simulink library "Simscape_Gimbals__Lib"  (R2025b)
settings: Solver=VariableStepAuto  StartTime=0.0  StopTime=10.0  RelTol=1e-3
undefined symbols (not defined in the file or in its folder): axisCmdType, baseAccEcho, baseRatesEcho, cmdTypes, dt, Motion, nFrames, Support, tFrame, tMotion, yawVec
libraries: nesl_utility x40, fl_lib x18, $bdroot x9, sm_lib x6, simulink_extras x6, simulink x1
(part 1 of 2)
settings Model: Creator=leoni  LastModifiedBy=Leonid

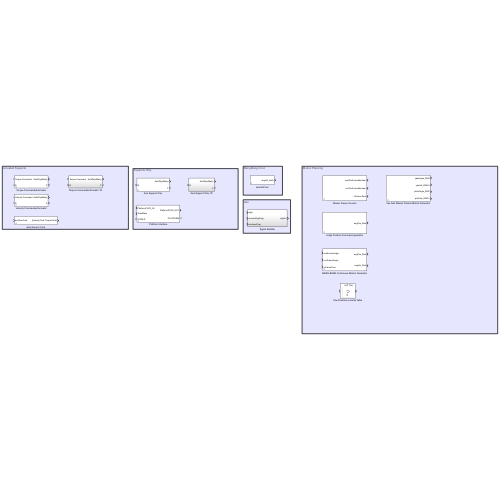
[thumbnail: Simulink's stored preview of the top-level diagram]
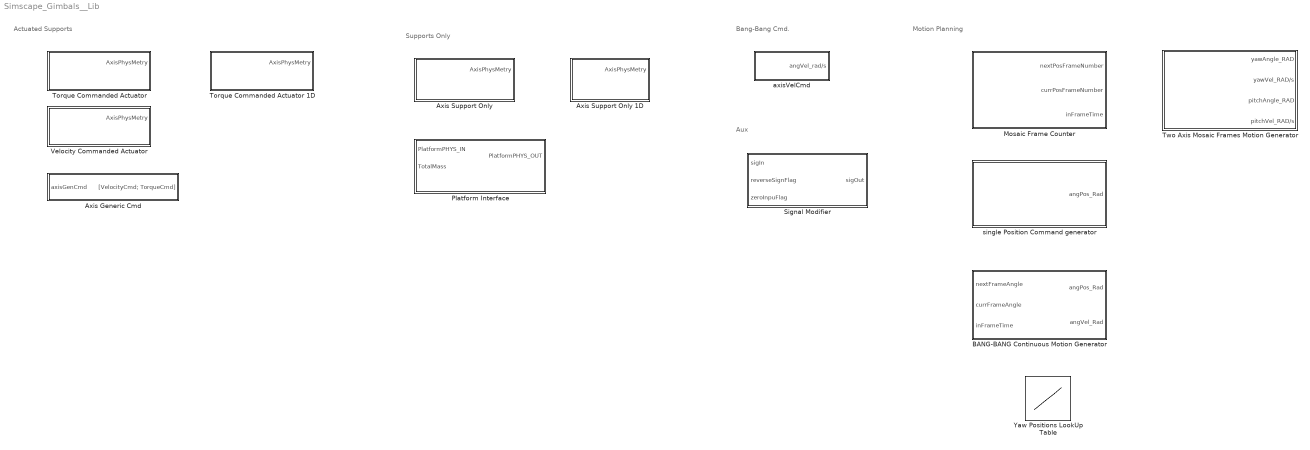
== system Simscape_Gimbals__Lib ==
  note: Aux
  note: Bang-Bang Cmd.
  note: Supports Only
  note: Actuated Supports
  note: Motion Planning
  Axis Generic Cmd : Subsystem  mask{AxisCmdType=axisCmdType}
      mask prompts: AxisCmdType "Axis Command Type"
  Axis Support Only : Subsystem  mask{bearingProps=0, noDist=on}
      mask prompts: bearingProps "Bearing Properties"; noDist "No Disturbances"
  Axis Support Only 1D : Subsystem
  BANG-BANG Continuous Motion Generator : Subsystem  mask{tMotion=tMotion, tFrame=tFrame}
      mask prompts: tMotion "Motion Time [s]"; tFrame "Frame Time [s]"
      mask DialogControl ParameterGroupVar Prompt: Bang-Bang
  Mosaic Frame Counter : Subsystem  mask{tFrame=tFrame, dt=dt, nFrames=0}
      mask prompts: tFrame "Frame time [s]"; dt "Sim resolution [s]"; nFrames "Number of Frames"
  Platform Interface : Subsystem  mask{mappingX=X, reverseX=off, mappingY=X, reverseY=off, mappingZ=X, reverseZ=off, noBaseMotion=off}
      mask prompts: mappingX "Map System X to World"; reverseX "Reverse X Direction"; mappingY "Map System Y to World"; reverseY "Reverse Y Direction"; mappingZ "Map System Z to World"; reverseZ "Reverse Z Direction"; noBaseMotion "No Base Motion"
      mask DialogControl ParameterGroupVar Prompt: CS MAPPING
      mask DialogControl Container3 Prompt: Simplifications
  Signal Modifier : Subsystem
  Torque Commanded Actuator : Subsystem  mask{bearingProps=0, harnessConstant=0, noDist=on}
      mask prompts: bearingProps "Bearing Properties"; harnessConstant "Harness Constant [mNm/rad]"; noDist "No Disturbances"
  Torque Commanded Actuator 1D : Subsystem
  Two Axis Mosaic Frames Motion Generator : Subsystem  mask{dt=0, tFrame=0, tMotion=0, nFrames=0, yawVec_DEG=0, pitchVec_DEG=0}
      mask prompts: dt "Simulation Time Resolution [s]"; tFrame "Single Frame Duration [s]"; tMotion "In Frame Motion Duration [s]"; nFrames "Total Number Of Frames"; yawVec_DEG "Yaw Axis Angle Sequence [DEG}"; pitchVec_DEG "PitchAxis Angle Sequence [DEG]"
      mask DialogControl ParameterGroupVar Prompt: Motion Time Properties
      mask DialogControl Container3 Prompt: Motion Angles
  Velocity Commanded Actuator : Subsystem  mask{bearingProps=0, harnessConstant=0}
      mask prompts: bearingProps "Bearing Properties"; harnessConstant "Harness Constant [mNm/rad]"
  Yaw Positions LookUp Table : Lookup_n-D  NumberOfTableDimensions=1  BreakpointsForDimension1=1:nFrames  Table=yawVec  InternalRulePriority=Speed  RndMeth=Simplest
  axisVelCmd : Subsystem  mask{travel=0.0, tMotion=0.0, tStart=0}
      mask prompts: travel "Travel Angle [deg]"; tMotion "Motion Duration [ms]"; tStart "Starting Time [s]"
      mask DialogControl ParameterGroupVar Prompt: Bang-Bang
  single Position Command generator : Subsystem  mask{Angle=15, Time=70}
      mask prompts: Angle "Travel Angle [deg]"; Time "Travel Time [ms]"
      mask DialogControl ParameterGroupVar Prompt: Bang-Bang

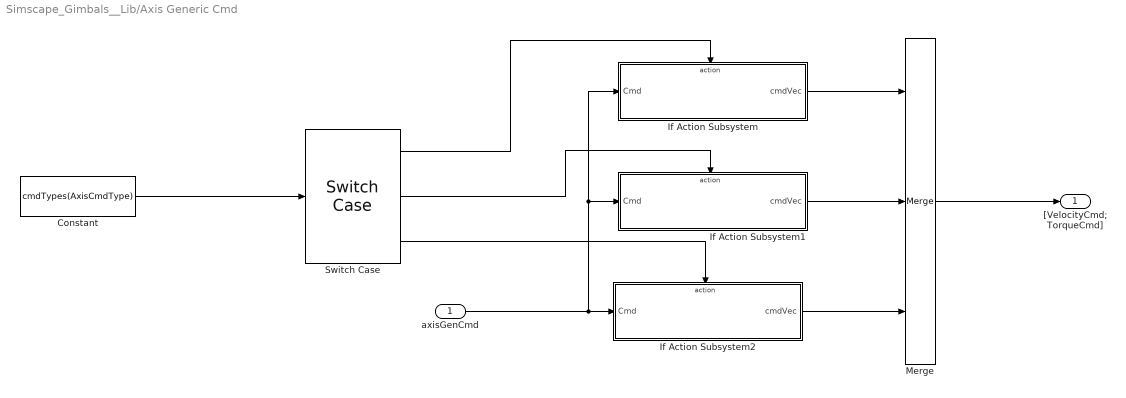
== system Simscape_Gimbals__Lib/Axis Generic Cmd ==
  axisGenCmd : Inport
  Constant : Constant  Value=cmdTypes(AxisCmdType)  OutDataTypeStr=Enum: cmdTypes
  If Action Subsystem : Subsystem  TreatAsAtomicUnit=on
  If Action Subsystem1 : Subsystem  TreatAsAtomicUnit=on
  If Action Subsystem2 : Subsystem  TreatAsAtomicUnit=on
  Merge : Merge  Inputs=3
  Switch Case : SwitchCase  CaseConditions={cmdTypes(1), cmdTypes(2)}
  "[VelocityCmd; TorqueCmd]" : Outport
  wires:
  Switch Case/1 -> If Action Subsystem/Action
  Switch Case/2 -> If Action Subsystem1/Action
  Switch Case/3 -> If Action Subsystem2/Action
  If Action Subsystem2/1(cmdVec) -> Merge/3
  If Action Subsystem1/1(cmdVec) -> Merge/2
  If Action Subsystem/1(cmdVec) -> Merge/1
  Merge/1 -> "[VelocityCmd; TorqueCmd]"/1
  axisGenCmd/1 -> If Action Subsystem/1(Cmd), If Action Subsystem1/1(Cmd), If Action Subsystem2/1(Cmd)
  Constant/1 -> Switch Case/1

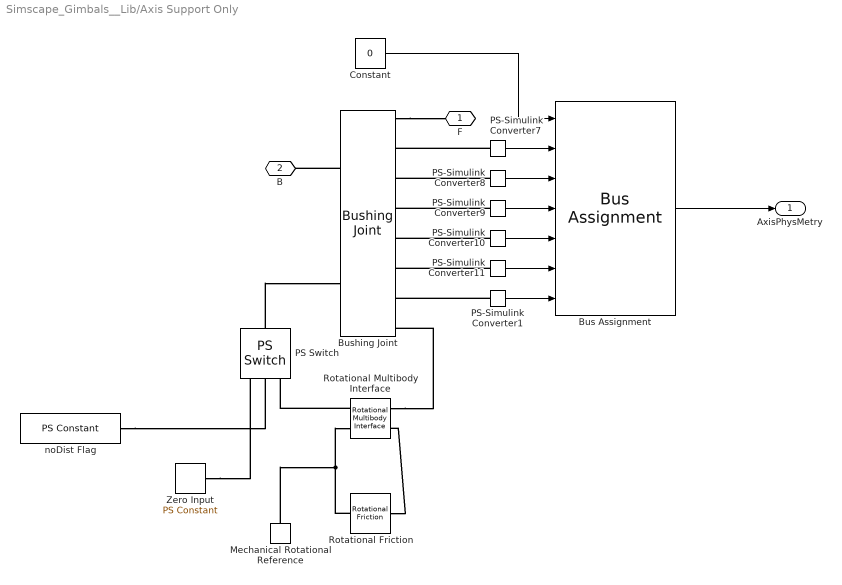
== system Simscape_Gimbals__Lib/Axis Support Only ==
  Bus Assignment : BusAssignment  AssignedSignals=Support.pX,Support.pY,Support.pZ,Support.qX,Support.qY,Motion.AxisPosition
  Bushing Joint : sm_lib/Joints/Bushing Joint  JointMode=Normal  CompositeWrenchDir=FollowerOnBase  CompositeWrenchFrame=BaseFrame  SenseConstraintForce=off  SenseConstraintTorque=off  SenseTotalForce=off  SenseTotalTorque=off  PxPositionTargetSpecify=off  PxPositionTargetPriority=High  PxPositionTargetValue=0  PxPositionTargetValueUnits=m  PxVelocityTargetSpecify=off  PxVelocityTargetPriority=High  PxVelocityTargetValue=0  PxVelocityTargetValueUnits=m/s  PxEquilibriumPosition=0.0  PxEquilibriumPositionUnits=mm  PxSpringStiffness=bearingProps.Krad  PxSpringStiffnessUnits=N/mm  PxDampingCoefficient=bearingProps.Crad  PxDampingCoefficientUnits=N/(m/s)  PxLowerLimitSpecify=off  PxLowerLimitBound=-1  PxLowerLimitBoundUnits=m  PxLowerLimitStiffness=1e6  PxLowerLimitStiffnessUnits=N/m  PxLowerLimitDamping=1e3  PxLowerLimitDampingUnits=N/(m/s)  PxLowerLimitTransitionRegionWidth=1e-4  PxLowerLimitTransitionRegionWidthUnits=m  PxUpperLimitSpecify=off  PxUpperLimitBound=1  PxUpperLimitBoundUnits=m  PxUpperLimitStiffness=1e6  PxUpperLimitStiffnessUnits=N/m  PxUpperLimitDamping=1e3  PxUpperLimitDampingUnits=N/(m/s)  PxUpperLimitTransitionRegionWidth=1e-4  PxUpperLimitTransitionRegionWidthUnits=m  PxTorqueActuationMode=NoTorque  PxMotionActuationMode=ComputedMotion  PxSensePosition=on  PxSenseVelocity=off  PxSenseAcceleration=off  PxSenseTorqueForce=off  PxSenseLowerLimitTorqueForce=off  PxSenseUpperLimitTorqueForce=off  PyPositionTargetSpecify=off  PyPositionTargetPriority=High  PyPositionTargetValue=0  PyPositionTargetValueUnits=m  PyVelocityTargetSpecify=off  PyVelocityTargetPriority=High  PyVelocityTargetValue=0  PyVelocityTargetValueUnits=m/s  PyEquilibriumPosition=0  PyEquilibriumPositionUnits=m  PySpringStiffness=bearingProps.Krad  PySpringStiffnessUnits=N/mm  PyDampingCoefficient=bearingProps.Crad  PyDampingCoefficientUnits=N/(m/s)  PyLowerLimitSpecify=off  PyLowerLimitBound=-1  PyLowerLimitBoundUnits=m  PyLowerLimitStiffness=1e6  PyLowerLimitStiffnessUnits=N/m  PyLowerLimitDamping=1e3  PyLowerLimitDampingUnits=N/(m/s)  PyLowerLimitTransitionRegionWidth=1e-4  PyLowerLimitTransitionRegionWidthUnits=m  PyUpperLimitSpecify=off  PyUpperLimitBound=1  PyUpperLimitBoundUnits=m  PyUpperLimitStiffness=1e6  PyUpperLimitStiffnessUnits=N/m  PyUpperLimitDamping=1e3  PyUpperLimitDampingUnits=N/(m/s)  PyUpperLimitTransitionRegionWidth=1e-4  PyUpperLimitTransitionRegionWidthUnits=m  PyTorqueActuationMode=NoTorque  PyMotionActuationMode=ComputedMotion  PySensePosition=on  PySenseVelocity=off  PySenseAcceleration=off  PySenseTorqueForce=off  PySenseLowerLimitTorqueForce=off  PySenseUpperLimitTorqueForce=off  PzPositionTargetSpecify=off  PzPositionTargetPriority=High  PzPositionTargetValue=0  PzPositionTargetValueUnits=m  PzVelocityTargetSpecify=off  PzVelocityTargetPriority=High  PzVelocityTargetValue=0  PzVelocityTargetValueUnits=m/s  PzEquilibriumPosition=0.0  PzEquilibriumPositionUnits=mm  PzSpringStiffness=bearingProps.Kax  PzSpringStiffnessUnits=N/mm  PzDampingCoefficient=bearingProps.Cax  PzDampingCoefficientUnits=N/(m/s)  PzLowerLimitSpecify=off  PzLowerLimitBound=-1  PzLowerLimitBoundUnits=m  PzLowerLimitStiffness=1e6  PzLowerLimitStiffnessUnits=N/m  PzLowerLimitDamping=1e3  PzLowerLimitDampingUnits=N/(m/s)  PzLowerLimitTransitionRegionWidth=1e-4  PzLowerLimitTransitionRegionWidthUnits=m  PzUpperLimitSpecify=off  PzUpperLimitBound=1  PzUpperLimitBoundUnits=m  PzUpperLimitStiffness=1e6  PzUpperLimitStiffnessUnits=N/m  PzUpperLimitDamping=1e3  PzUpperLimitDampingUnits=N/(m/s)  PzUpperLimitTransitionRegionWidth=1e-4  PzUpperLimitTransitionRegionWidthUnits=m  PzTorqueActuationMode=NoTorque  PzMotionActuationMode=ComputedMotion  PzSensePosition=on  PzSenseVelocity=off  PzSenseAcceleration=off  PzSenseTorqueForce=off  PzSenseLowerLimitTorqueForce=off  PzSenseUpperLimitTorqueForce=off  RxPositionTargetSpecify=off  RxPositionTargetPriority=High  RxPositionTargetValue=0  RxPositionTargetValueUnits=deg  RxVelocityTargetSpecify=off  RxVelocityTargetPriority=High  RxVelocityTargetValue=0  RxVelocityTargetValueUnits=deg/s  RxEquilibriumPosition=0.0  RxEquilibriumPositionUnits=deg  RxSpringStiffness=bearingProps.Kang  RxSpringStiffnessUnits=N*m/rad  RxDampingCoefficient=bearingProps.Cang  RxDampingCoefficientUnits=N*m*s/rad  RxLowerLimitSpecify=off  RxLowerLimitBound=-90  RxLowerLimitBoundUnits=deg  RxLowerLimitStiffness=1e4  RxLowerLimitStiffnessUnits=N*m/deg  RxLowerLimitDamping=10  RxLowerLimitDampingUnits=N*m/(deg/s)  RxLowerLimitTransitionRegionWidth=0.1  RxLowerLimitTransitionRegionWidthUnits=deg  RxUpperLimitSpecify=off  RxUpperLimitBound=90  RxUpperLimitBoundUnits=deg  RxUpperLimitStiffness=1e4  RxUpperLimitStiffnessUnits=N*m/deg  RxUpperLimitDamping=10  RxUpperLimitDampingUnits=N*m/(deg/s)  RxUpperLimitTransitionRegionWidth=0.1  RxUpperLimitTransitionRegionWidthUnits=deg  RxTorqueActuationMode=NoTorque  RxMotionActuationMode=ComputedMotion  RxSensePosition=on  RxSenseVelocity=off  RxSenseAcceleration=off  RxSenseTorqueForce=off  RxSenseLowerLimitTorqueForce=off  RxSenseUpperLimitTorqueForce=off  RyPositionTargetSpecify=off  RyPositionTargetPriority=High  RyPositionTargetValue=0  RyPositionTargetValueUnits=deg  RyVelocityTargetSpecify=off  RyVelocityTargetPriority=High  RyVelocityTargetValue=0  RyVelocityTargetValueUnits=deg/s  RyEquilibriumPosition=0.0  RyEquilibriumPositionUnits=deg  RySpringStiffness=bearingProps.Kang  RySpringStiffnessUnits=N*m/rad  RyDampingCoefficient=bearingProps.Cang  RyDampingCoefficientUnits=N*m*s/rad  RyLowerLimitSpecify=off  RyLowerLimitBound=-90  RyLowerLimitBoundUnits=deg  RyLowerLimitStiffness=1e4  RyLowerLimitStiffnessUnits=N*m/deg  RyLowerLimitDamping=10  RyLowerLimitDampingUnits=N*m/(deg/s)  RyLowerLimitTransitionRegionWidth=0.1  RyLowerLimitTransitionRegionWidthUnits=deg  RyUpperLimitSpecify=off  RyUpperLimitBound=90  RyUpperLimitBoundUnits=deg  RyUpperLimitStiffness=1e4  RyUpperLimitStiffnessUnits=N*m/deg  RyUpperLimitDamping=10  RyUpperLimitDampingUnits=N*m/(deg/s)  RyUpperLimitTransitionRegionWidth=0.1  RyUpperLimitTransitionRegionWidthUnits=deg  RyTorqueActuationMode=NoTorque  RyMotionActuationMode=ComputedMotion  RySensePosition=on  RySenseVelocity=off  RySenseAcceleration=off  RySenseTorqueForce=off  RySenseLowerLimitTorqueForce=off  RySenseUpperLimitTorqueForce=off  RzPositionTargetSpecify=off  RzPositionTargetPriority=High  RzPositionTargetValue=0  RzPositionTargetValueUnits=deg  RzVelocityTargetSpecify=off  RzVelocityTargetPriority=High  RzVelocityTargetValue=0  RzVelocityTargetValueUnits=deg/s  RzEquilibriumPosition=0  RzEquilibriumPositionUnits=deg  RzSpringStiffness=0  RzSpringStiffnessUnits=N*m/deg  RzDampingCoefficient=0  RzDampingCoefficientUnits=N*m/(deg/s)  RzLowerLimitSpecify=off  RzLowerLimitBound=-90  RzLowerLimitBoundUnits=deg  RzLowerLimitStiffness=1e4  RzLowerLimitStiffnessUnits=N*m/deg  RzLowerLimitDamping=10  RzLowerLimitDampingUnits=N*m/(deg/s)  RzLowerLimitTransitionRegionWidth=0.1  RzLowerLimitTransitionRegionWidthUnits=deg  RzUpperLimitSpecify=off  RzUpperLimitBound=90  RzUpperLimitBoundUnits=deg  RzUpperLimitStiffness=1e4  RzUpperLimitStiffnessUnits=N*m/deg  RzUpperLimitDamping=10  RzUpperLimitDampingUnits=N*m/(deg/s)  RzUpperLimitTransitionRegionWidth=0.1  RzUpperLimitTransitionRegionWidthUnits=deg  RzTorqueActuationMode=InputTorque  RzMotionActuationMode=ComputedMotion  RzSensePosition=on  RzSenseVelocity=on  RzSenseAcceleration=off  RzSenseTorqueForce=off  RzSenseLowerLimitTorqueForce=off  RzSenseUpperLimitTorqueForce=off
  Constant : Constant  Value=0  OutDataTypeStr=Bus: AxisMetry
  Mechanical Rotational Reference : fl_lib/Mechanical/Rotational Elements/Mechanical Rotational Reference
  PS Switch : fl_lib/Physical Signals/Nonlinear Operators/PS Switch  Threshold=0.5  ZeroCross=true
      settings: InternalSimscapePortConfiguration="{\"Bottom\":[],\"Left\":[{\"id\":\"I1\",\"label\":\"\",\"type\":\"input\"},{\"id\":\"I2\",\"label\":\"\",\"type\":\"input\"},{\"id\":\"I3\",\"label\":\"\",\"type\":\"input\"}],\"Right\":[{\"id\":\"O\",\"label\":\"\",\"type\":\"output\"}],\"Top\":[]}"
  PS-Simulink Converter1 : nesl_utility/PS-Simulink Converter  PhysicalDomain=network_engine_domain  SubClassName=ps_output  LeftPortType=input  RightPortType=output  PseudoPeriodic=off  Frequencies=[]  VectorFormat=inherit  Unit=rad  AffineConversion=off
  PS-Simulink Converter10 : nesl_utility/PS-Simulink Converter  PhysicalDomain=network_engine_domain  SubClassName=ps_output  LeftPortType=input  RightPortType=output  PseudoPeriodic=off  Frequencies=[]  VectorFormat=inherit  Unit=rad  AffineConversion=off
  PS-Simulink Converter11 : nesl_utility/PS-Simulink Converter  PhysicalDomain=network_engine_domain  SubClassName=ps_output  LeftPortType=input  RightPortType=output  PseudoPeriodic=off  Frequencies=[]  VectorFormat=inherit  Unit=rad  AffineConversion=off
  PS-Simulink Converter7 : nesl_utility/PS-Simulink Converter  PhysicalDomain=network_engine_domain  SubClassName=ps_output  LeftPortType=input  RightPortType=output  PseudoPeriodic=off  Frequencies=[]  VectorFormat=inherit  Unit=m  AffineConversion=off
  PS-Simulink Converter8 : nesl_utility/PS-Simulink Converter  PhysicalDomain=network_engine_domain  SubClassName=ps_output  LeftPortType=input  RightPortType=output  PseudoPeriodic=off  Frequencies=[]  VectorFormat=inherit  Unit=m  AffineConversion=off
  PS-Simulink Converter9 : nesl_utility/PS-Simulink Converter  PhysicalDomain=network_engine_domain  SubClassName=ps_output  LeftPortType=input  RightPortType=output  PseudoPeriodic=off  Frequencies=[]  VectorFormat=inherit  Unit=m  AffineConversion=off
  Rotational Friction : fl_lib/Mechanical/Rotational Elements/Rotational Friction  brkwy_trq=bearingProps.Tf*1.4 m*mN  brkwy_vel=0.1 rad/s  Col_trq=bearingProps.Tf m*mN  visc_coef=0.0 N*m*s/rad  w_specify=off  w_priority=None  w=0 rad/s  w_nominal_specify=off  w_nominal_value=1  w_nominal_unit=rad/s  t_specify=off  t_priority=None  t=0 N*m  t_nominal_specify=off  t_nominal_value=1  t_nominal_unit=N*m
  Rotational Multibody Interface : fl_lib/Mechanical/Multibody Interfaces/Rotational Multibody Interface
  Zero Input : fl_lib/Physical Signals/Sources/PS Constant  constant=0 N*m
  noDist Flag : fl_lib/Physical Signals/Sources/PS Constant  constant=noDist
  F : PMIOPort  Side=Right
  B : PMIOPort  Port=2  Side=Left
  AxisPhysMetry : Outport
  wires:
  Constant/1 -> Bus Assignment/1
  Bus Assignment/1 -> AxisPhysMetry/1
  PS-Simulink Converter9/1 -> Bus Assignment/4
  PS-Simulink Converter10/1 -> Bus Assignment/5
  PS-Simulink Converter11/1 -> Bus Assignment/6
  PS-Simulink Converter8/1 -> Bus Assignment/3
  PS-Simulink Converter7/1 -> Bus Assignment/2
  PS-Simulink Converter1/1 -> Bus Assignment/7
  connections:
  Rotational Friction/LConn1 -- Rotational Multibody Interface/RConn2
  Mechanical Rotational Reference/LConn1 -- Rotational Friction/RConn1 -- Rotational Multibody Interface/LConn2
  PS-Simulink Converter11/LConn1 -- Bushing Joint/RConn6
  PS-Simulink Converter9/LConn1 -- Bushing Joint/RConn4
  PS-Simulink Converter10/LConn1 -- Bushing Joint/RConn5
  Rotational Multibody Interface/RConn1 -- Bushing Joint/RConn8
  PS-Simulink Converter7/LConn1 -- Bushing Joint/RConn2
  PS-Simulink Converter1/LConn1 -- Bushing Joint/RConn7
  Bushing Joint/RConn1 -- F/RConn1
  Bushing Joint/LConn1 -- B/RConn1
  PS-Simulink Converter8/LConn1 -- Bushing Joint/RConn3
  Rotational Multibody Interface/LConn1 -- PS Switch/LConn3
  PS Switch/RConn1 -- Bushing Joint/LConn2
  noDist Flag/RConn1 -- PS Switch/LConn2
  Zero Input/RConn1 -- PS Switch/LConn1

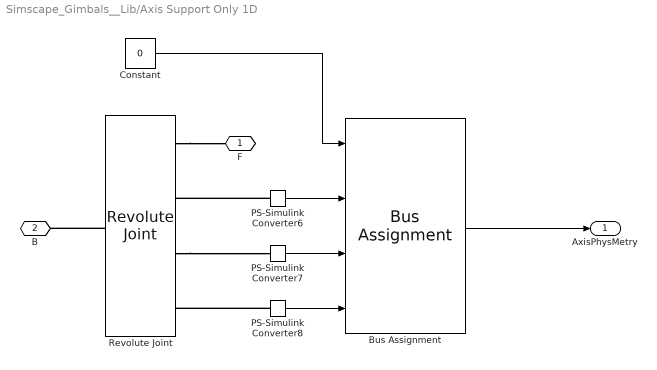
== system Simscape_Gimbals__Lib/Axis Support Only 1D ==
  Bus Assignment : BusAssignment  AssignedSignals=Motion.AxisPosition,Motion.AxisVelocity,Motion.AxisTorque
  Constant : Constant  Value=0  OutDataTypeStr=Bus: AxisMetry
  PS-Simulink Converter6 : nesl_utility/PS-Simulink Converter  PhysicalDomain=network_engine_domain  SubClassName=ps_output  LeftPortType=input  RightPortType=output  PseudoPeriodic=off  Frequencies=[]  VectorFormat=inherit  Unit=rad  AffineConversion=off
  PS-Simulink Converter7 : nesl_utility/PS-Simulink Converter  PhysicalDomain=network_engine_domain  SubClassName=ps_output  LeftPortType=input  RightPortType=output  PseudoPeriodic=off  Frequencies=[]  VectorFormat=inherit  Unit=rad/s  AffineConversion=off
  PS-Simulink Converter8 : nesl_utility/PS-Simulink Converter  PhysicalDomain=network_engine_domain  SubClassName=ps_output  LeftPortType=input  RightPortType=output  PseudoPeriodic=off  Frequencies=[]  VectorFormat=inherit  Unit=N*m  AffineConversion=off
  Revolute Joint : sm_lib/Joints/Revolute Joint  JointMode=Normal  CompositeWrenchDir=FollowerOnBase  CompositeWrenchFrame=BaseFrame  SenseConstraintForce=off  SenseConstraintTorque=off  SenseTotalForce=off  SenseTotalTorque=off  PositionTargetSpecify=off  PositionTargetPriority=High  PositionTargetValue=0  PositionTargetValueUnits=deg  VelocityTargetSpecify=off  VelocityTargetPriority=High  VelocityTargetValue=0  VelocityTargetValueUnits=deg/s  EquilibriumPosition=0  EquilibriumPositionUnits=deg  SpringStiffness=0  SpringStiffnessUnits=N*m/deg  DampingCoefficient=0  DampingCoefficientUnits=N*m/(deg/s)  LowerLimitSpecify=off  LowerLimitBound=-90  LowerLimitBoundUnits=deg  LowerLimitStiffness=1e4  LowerLimitStiffnessUnits=N*m/deg  LowerLimitDamping=10  LowerLimitDampingUnits=N*m/(deg/s)  LowerLimitTransitionRegionWidth=0.1  LowerLimitTransitionRegionWidthUnits=deg  UpperLimitSpecify=off  UpperLimitBound=90  UpperLimitBoundUnits=deg  UpperLimitStiffness=1e4  UpperLimitStiffnessUnits=N*m/deg  UpperLimitDamping=10  UpperLimitDampingUnits=N*m/(deg/s)  UpperLimitTransitionRegionWidth=0.1  UpperLimitTransitionRegionWidthUnits=deg  TorqueActuationMode=NoTorque  MotionActuationMode=ComputedMotion  SensePosition=on  SenseVelocity=on  SenseAcceleration=off  SenseTorqueForce=on  SenseLowerLimitTorqueForce=off  SenseUpperLimitTorqueForce=off
  F : PMIOPort  Side=Right
  B : PMIOPort  Port=2  Side=Left
  AxisPhysMetry : Outport
  wires:
  Constant/1 -> Bus Assignment/1
  PS-Simulink Converter6/1 -> Bus Assignment/2
  PS-Simulink Converter7/1 -> Bus Assignment/3
  PS-Simulink Converter8/1 -> Bus Assignment/4
  Bus Assignment/1 -> AxisPhysMetry/1
  connections:
  Revolute Joint/LConn1 -- B/RConn1
  Revolute Joint/RConn1 -- F/RConn1
  PS-Simulink Converter6/LConn1 -- Revolute Joint/RConn2
  Revolute Joint/RConn3 -- PS-Simulink Converter7/LConn1
  PS-Simulink Converter8/LConn1 -- Revolute Joint/RConn4

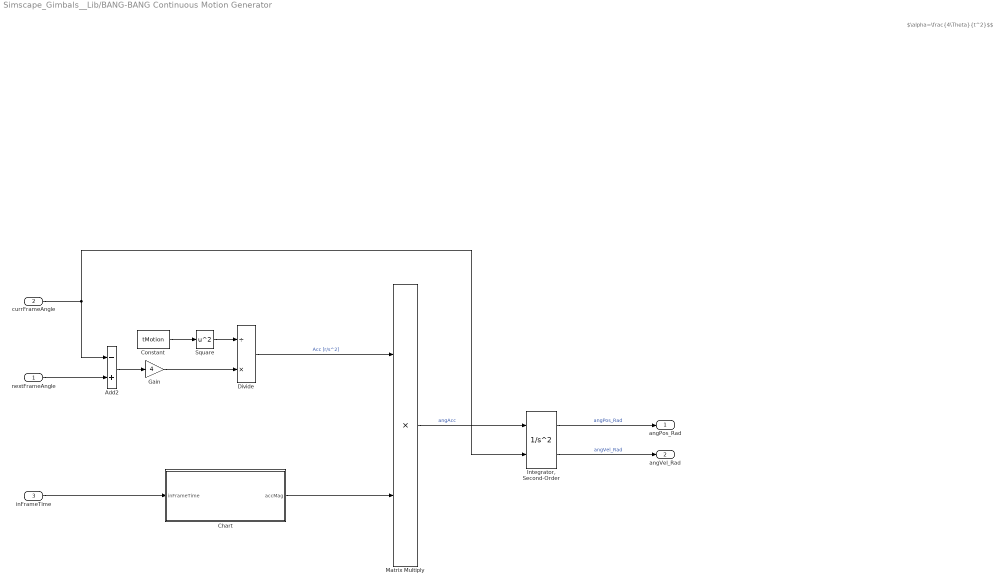
== system Simscape_Gimbals__Lib/BANG-BANG Continuous Motion Generator ==
  note: $\alpha=\frac{4\Theta}{t^2}$$
  nextFrameAngle : Inport
  currFrameAngle : Inport  Port=2
  inFrameTime : Inport  Port=3
  Add2 : Sum  Inputs=-+
  Chart : Stateflow chart  TreatAsAtomicUnit=on
  Constant : Constant  Value=tMotion
  Divide : Product  Inputs=/*
  Gain : Gain  Gain=4
  "Integrator, Second-Order" : SecondOrderIntegrator  ICSourceX=external
  Matrix Multiply : Product
  Square : Math  Operator=square
  angPos_Rad : Outport
  angVel_Rad : Outport  Port=2
  wires:
  Chart/1(accMag) -> Matrix Multiply/2
  Divide/1 -> Matrix Multiply/1  "Acc [r/s^2]"
  Matrix Multiply/1 -> "Integrator, Second-Order"/1  "angAcc"
  "Integrator, Second-Order"/1 -> angPos_Rad/1  "angPos_Rad"
  "Integrator, Second-Order"/2 -> angVel_Rad/1  "angVel_Rad"
  Constant/1 -> Square/1
  Gain/1 -> Divide/2
  Square/1 -> Divide/1
  inFrameTime/1 -> Chart/1(inFrameTime)
  Add2/1 -> Gain/1
  currFrameAngle/1 -> Add2/1, "Integrator, Second-Order"/2
  nextFrameAngle/1 -> Add2/2

== system Simscape_Gimbals__Lib/Mosaic Frame Counter ==
  Clock : Clock
  Compare To Constant : simulink/Logic and Bit Operations/Compare To Constant  relop=<=  const=dt*2  OutDataTypeStr=boolean
  Mod : Math  Operator=mod
  Triggered Subsystem : Subsystem  TreatAsAtomicUnit=on
  frame time : Constant  Value=tFrame
  nextPosFrameNumber : Outport
  currPosFrameNumber : Outport  Port=2
  inFrameTime : Outport  Port=3
  wires:
  Triggered Subsystem/1(currCMD) -> nextPosFrameNumber/1
  Mod/1 -> inFrameTime/1, Compare To Constant/1
  frame time/1 -> Mod/2
  Compare To Constant/1 -> Triggered Subsystem/Trigger
  Clock/1 -> Mod/1
  Triggered Subsystem/2(currPOS) -> currPosFrameNumber/1

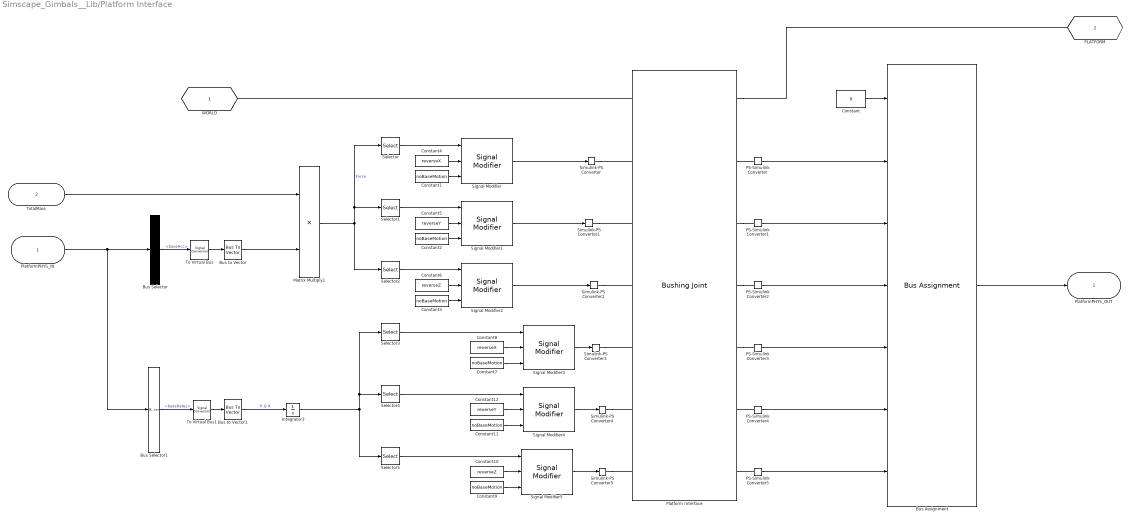
== system Simscape_Gimbals__Lib/Platform Interface ==
  PlatformPHYS_IN : Inport  OutDataTypeStr=Bus: PHYS_IN
  TotalMass : Inport  Port=2
  Bus Assignment : BusAssignment  AssignedSignals=baseAccEcho.aX,baseAccEcho.aY,baseAccEcho.aZ,baseRatesEcho.wX,baseRatesEcho.wY,baseRatesEcho.wZ
  Bus Selector : BusSelector  OutputSignals=baseAcc
  Bus Selector1 : BusSelector  OutputSignals=baseRates
  Bus to Vector : BusToVector
  Bus to Vector1 : BusToVector
  Constant : Constant  Value=0  OutDataTypeStr=Bus: PHYS_OUT  SampleTime=-1
  Constant{1..3,7,9,11} (6 alike) : Constant  Value=noBaseMotion
  Constant10 : Constant  Value=reverseZ
  Constant12 : Constant  Value=reverseY
  Constant4 : Constant  Value=reverseX
  Constant5 : Constant  Value=reverseY
  Constant6 : Constant  Value=reverseZ
  Constant8 : Constant  Value=reverseX
  Integrator3 : Integrator
  Matrix Multiply1 : Product
  PS-Simulink Converter : nesl_utility/PS-Simulink Converter  PhysicalDomain=network_engine_domain  SubClassName=ps_output  LeftPortType=input  RightPortType=output  PseudoPeriodic=off  Frequencies=[]  VectorFormat=inherit  Unit=m/s^2  AffineConversion=off
  PS-Simulink Converter1 : nesl_utility/PS-Simulink Converter  PhysicalDomain=network_engine_domain  SubClassName=ps_output  LeftPortType=input  RightPortType=output  PseudoPeriodic=off  Frequencies=[]  VectorFormat=inherit  Unit=m/s^2  AffineConversion=off
  PS-Simulink Converter2 : nesl_utility/PS-Simulink Converter  PhysicalDomain=network_engine_domain  SubClassName=ps_output  LeftPortType=input  RightPortType=output  PseudoPeriodic=off  Frequencies=[]  VectorFormat=inherit  Unit=m/s^2  AffineConversion=off
  PS-Simulink Converter3 : nesl_utility/PS-Simulink Converter  PhysicalDomain=network_engine_domain  SubClassName=ps_output  LeftPortType=input  RightPortType=output  PseudoPeriodic=off  Frequencies=[]  VectorFormat=inherit  Unit=rad/s  AffineConversion=off
  PS-Simulink Converter4 : nesl_utility/PS-Simulink Converter  PhysicalDomain=network_engine_domain  SubClassName=ps_output  LeftPortType=input  RightPortType=output  PseudoPeriodic=off  Frequencies=[]  VectorFormat=inherit  Unit=rad/s  AffineConversion=off
  PS-Simulink Converter5 : nesl_utility/PS-Simulink Converter  PhysicalDomain=network_engine_domain  SubClassName=ps_output  LeftPortType=input  RightPortType=output  PseudoPeriodic=off  Frequencies=[]  VectorFormat=inherit  Unit=rad/s  AffineConversion=off
  Platform Interface : sm_lib/Joints/Bushing Joint  JointMode=Normal  CompositeWrenchDir=FollowerOnBase  CompositeWrenchFrame=BaseFrame  SenseConstraintForce=off  SenseConstraintTorque=off  SenseTotalForce=off  SenseTotalTorque=off  PxPositionTargetSpecify=off  PxPositionTargetPriority=High  PxPositionTargetValue=0  PxPositionTargetValueUnits=m  PxVelocityTargetSpecify=off  PxVelocityTargetPriority=High  PxVelocityTargetValue=0  PxVelocityTargetValueUnits=m/s  PxEquilibriumPosition=0  PxEquilibriumPositionUnits=m  PxSpringStiffness=0  PxSpringStiffnessUnits=N/m  PxDampingCoefficient=0  PxDampingCoefficientUnits=N/(m/s)  PxLowerLimitSpecify=off  PxLowerLimitBound=-1  PxLowerLimitBoundUnits=m  PxLowerLimitStiffness=1e6  PxLowerLimitStiffnessUnits=N/m  PxLowerLimitDamping=1e3  PxLowerLimitDampingUnits=N/(m/s)  PxLowerLimitTransitionRegionWidth=1e-4  PxLowerLimitTransitionRegionWidthUnits=m  PxUpperLimitSpecify=off  PxUpperLimitBound=1  PxUpperLimitBoundUnits=m  PxUpperLimitStiffness=1e6  PxUpperLimitStiffnessUnits=N/m  PxUpperLimitDamping=1e3  PxUpperLimitDampingUnits=N/(m/s)  PxUpperLimitTransitionRegionWidth=1e-4  PxUpperLimitTransitionRegionWidthUnits=m  PxTorqueActuationMode=InputTorque  PxMotionActuationMode=ComputedMotion  PxSensePosition=off  PxSenseVelocity=off  PxSenseAcceleration=on  PxSenseTorqueForce=off  PxSenseLowerLimitTorqueForce=off  PxSenseUpperLimitTorqueForce=off  PyPositionTargetSpecify=off  PyPositionTargetPriority=High  PyPositionTargetValue=0  PyPositionTargetValueUnits=m  PyVelocityTargetSpecify=off  PyVelocityTargetPriority=High  PyVelocityTargetValue=0  PyVelocityTargetValueUnits=m/s  PyEquilibriumPosition=0  PyEquilibriumPositionUnits=m  PySpringStiffness=0  PySpringStiffnessUnits=N/m  PyDampingCoefficient=0  PyDampingCoefficientUnits=N/(m/s)  PyLowerLimitSpecify=off  PyLowerLimitBound=-1  PyLowerLimitBoundUnits=m  PyLowerLimitStiffness=1e6  PyLowerLimitStiffnessUnits=N/m  PyLowerLimitDamping=1e3  PyLowerLimitDampingUnits=N/(m/s)  PyLowerLimitTransitionRegionWidth=1e-4  PyLowerLimitTransitionRegionWidthUnits=m  PyUpperLimitSpecify=off  PyUpperLimitBound=1  PyUpperLimitBoundUnits=m  PyUpperLimitStiffness=1e6  PyUpperLimitStiffnessUnits=N/m  PyUpperLimitDamping=1e3  PyUpperLimitDampingUnits=N/(m/s)  PyUpperLimitTransitionRegionWidth=1e-4  PyUpperLimitTransitionRegionWidthUnits=m  PyTorqueActuationMode=InputTorque  PyMotionActuationMode=ComputedMotion  PySensePosition=off  PySenseVelocity=off  PySenseAcceleration=on  PySenseTorqueForce=off  PySenseLowerLimitTorqueForce=off  PySenseUpperLimitTorqueForce=off  PzPositionTargetSpecify=off  PzPositionTargetPriority=High  PzPositionTargetValue=0  PzPositionTargetValueUnits=m  PzVelocityTargetSpecify=off  PzVelocityTargetPriority=High  PzVelocityTargetValue=0  PzVelocityTargetValueUnits=m/s  PzEquilibriumPosition=0  PzEquilibriumPositionUnits=m  PzSpringStiffness=0  PzSpringStiffnessUnits=N/m  PzDampingCoefficient=0  PzDampingCoefficientUnits=N/(m/s)  PzLowerLimitSpecify=off  PzLowerLimitBound=-1  PzLowerLimitBoundUnits=m  PzLowerLimitStiffness=1e6  PzLowerLimitStiffnessUnits=N/m  PzLowerLimitDamping=1e3  PzLowerLimitDampingUnits=N/(m/s)  PzLowerLimitTransitionRegionWidth=1e-4  PzLowerLimitTransitionRegionWidthUnits=m  PzUpperLimitSpecify=off  PzUpperLimitBound=1  PzUpperLimitBoundUnits=m  PzUpperLimitStiffness=1e6  PzUpperLimitStiffnessUnits=N/m  PzUpperLimitDamping=1e3  PzUpperLimitDampingUnits=N/(m/s)  PzUpperLimitTransitionRegionWidth=1e-4  PzUpperLimitTransitionRegionWidthUnits=m  PzTorqueActuationMode=InputTorque  PzMotionActuationMode=ComputedMotion  PzSensePosition=off  PzSenseVelocity=off  PzSenseAcceleration=on  PzSenseTorqueForce=off  PzSenseLowerLimitTorqueForce=off  PzSenseUpperLimitTorqueForce=off  RxPositionTargetSpecify=off  RxPositionTargetPriority=High  RxPositionTargetValue=0  RxPositionTargetValueUnits=deg  RxVelocityTargetSpecify=off  RxVelocityTargetPriority=High  RxVelocityTargetValue=0  RxVelocityTargetValueUnits=deg/s  RxEquilibriumPosition=0  RxEquilibriumPositionUnits=deg  RxSpringStiffness=0  RxSpringStiffnessUnits=N*m/deg  RxDampingCoefficient=0  RxDampingCoefficientUnits=N*m/(deg/s)  RxLowerLimitSpecify=off  RxLowerLimitBound=-90  RxLowerLimitBoundUnits=deg  RxLowerLimitStiffness=1e4  RxLowerLimitStiffnessUnits=N*m/deg  RxLowerLimitDamping=10  RxLowerLimitDampingUnits=N*m/(deg/s)  RxLowerLimitTransitionRegionWidth=0.1  RxLowerLimitTransitionRegionWidthUnits=deg  RxUpperLimitSpecify=off  RxUpperLimitBound=90  RxUpperLimitBoundUnits=deg  RxUpperLimitStiffness=1e4  RxUpperLimitStiffnessUnits=N*m/deg  RxUpperLimitDamping=10  RxUpperLimitDampingUnits=N*m/(deg/s)  RxUpperLimitTransitionRegionWidth=0.1  RxUpperLimitTransitionRegionWidthUnits=deg  RxTorqueActuationMode=ComputedTorque  RxMotionActuationMode=InputMotion  RxSensePosition=off  RxSenseVelocity=on  RxSenseAcceleration=off  RxSenseTorqueForce=off  RxSenseLowerLimitTorqueForce=off  RxSenseUpperLimitTorqueForce=off  RyPositionTargetSpecify=off  RyPositionTargetPriority=High  RyPositionTargetValue=0  RyPositionTargetValueUnits=deg  RyVelocityTargetSpecify=off  RyVelocityTargetPriority=High  RyVelocityTargetValue=0  RyVelocityTargetValueUnits=deg/s  RyEquilibriumPosition=0  RyEquilibriumPositionUnits=deg  RySpringStiffness=0  RySpringStiffnessUnits=N*m/deg  RyDampingCoefficient=0  RyDampingCoefficientUnits=N*m/(deg/s)  RyLowerLimitSpecify=off  RyLowerLimitBound=-90  RyLowerLimitBoundUnits=deg  RyLowerLimitStiffness=1e4  RyLowerLimitStiffnessUnits=N*m/deg  RyLowerLimitDamping=10  RyLowerLimitDampingUnits=N*m/(deg/s)  RyLowerLimitTransitionRegionWidth=0.1  RyLowerLimitTransitionRegionWidthUnits=deg  RyUpperLimitSpecify=off  RyUpperLimitBound=90  RyUpperLimitBoundUnits=deg  RyUpperLimitStiffness=1e4  RyUpperLimitStiffnessUnits=N*m/deg  RyUpperLimitDamping=10  RyUpperLimitDampingUnits=N*m/(deg/s)  RyUpperLimitTransitionRegionWidth=0.1  RyUpperLimitTransitionRegionWidthUnits=deg  RyTorqueActuationMode=ComputedTorque  RyMotionActuationMode=InputMotion  RySensePosition=off  RySenseVelocity=on  RySenseAcceleration=off  RySenseTorqueForce=off  RySenseLowerLimitTorqueForce=off  RySenseUpperLimitTorqueForce=off  RzPositionTargetSpecify=off  RzPositionTargetPriority=High  RzPositionTargetValue=0  RzPositionTargetValueUnits=deg  RzVelocityTargetSpecify=off  RzVelocityTargetPriority=High  RzVelocityTargetValue=0  RzVelocityTargetValueUnits=deg/s  RzEquilibriumPosition=0  RzEquilibriumPositionUnits=deg  RzSpringStiffness=0  RzSpringStiffnessUnits=N*m/deg  RzDampingCoefficient=0  RzDampingCoefficientUnits=N*m/(deg/s)  RzLowerLimitSpecify=off  RzLowerLimitBound=-90  RzLowerLimitBoundUnits=deg  RzLowerLimitStiffness=1e4  RzLowerLimitStiffnessUnits=N*m/deg  RzLowerLimitDamping=10  RzLowerLimitDampingUnits=N*m/(deg/s)  RzLowerLimitTransitionRegionWidth=0.1  RzLowerLimitTransitionRegionWidthUnits=deg  RzUpperLimitSpecify=off  RzUpperLimitBound=90  RzUpperLimitBoundUnits=deg  RzUpperLimitStiffness=1e4  RzUpperLimitStiffnessUnits=N*m/deg  RzUpperLimitDamping=10  RzUpperLimitDampingUnits=N*m/(deg/s)  RzUpperLimitTransitionRegionWidth=0.1  RzUpperLimitTransitionRegionWidthUnits=deg  RzTorqueActuationMode=ComputedTorque  RzMotionActuationMode=InputMotion  RzSensePosition=off  RzSenseVelocity=on  RzSenseAcceleration=off  RzSenseTorqueForce=off  RzSenseLowerLimitTorqueForce=off  RzSenseUpperLimitTorqueForce=off
  Selector : Selector  InputPortWidth=3  IndexOptions=Index vector (dialog)  Indices=mappingX  OutputSizes=1
  Selector1 : Selector  InputPortWidth=3  IndexOptions=Index vector (dialog)  Indices=mappingY  OutputSizes=1
  Selector2 : Selector  InputPortWidth=3  IndexOptions=Index vector (dialog)  Indices=mappingZ  OutputSizes=1
  Selector3 : Selector  InputPortWidth=3  IndexOptions=Index vector (dialog)  Indices=mappingX  OutputSizes=1
  Selector4 : Selector  InputPortWidth=3  IndexOptions=Index vector (dialog)  Indices=mappingY  OutputSizes=1
  Selector5 : Selector  InputPortWidth=3  IndexOptions=Index vector (dialog)  Indices=mappingZ  OutputSizes=1
  Signal Modifier{,1..5} (6 alike) : $bdroot/Signal Modifier  SystemSampleTime=-1  VariantActivationTime=update diagram  EmptyChoice=off  PassThrough=off  PassThroughVariantControl=(default)  EmptyChoiceVariantControl=(default)  AllowFlexibleInterface=on  Latency=0  AutoFrameSizeCalculation=off
  Simulink-PS Converter : nesl_utility/Simulink-PS Converter  PhysicalDomain=network_engine_domain  SubClassName=ps_input  LeftPortType=input  RightPortType=output  PseudoPeriodic=off  Frequencies=[]  NoiseDistribution=none  NoiseParameters=[]  Unit=N  AffineConversion=off  FilteringAndDerivatives=provide  SimscapeFilterOrder=1  InputFilterTimeConstant=0.001  UdotUserProvided=0
  Simulink-PS Converter1 : nesl_utility/Simulink-PS Converter  PhysicalDomain=network_engine_domain  SubClassName=ps_input  LeftPortType=input  RightPortType=output  PseudoPeriodic=off  Frequencies=[]  NoiseDistribution=none  NoiseParameters=[]  Unit=N  AffineConversion=off  FilteringAndDerivatives=provide  SimscapeFilterOrder=1  InputFilterTimeConstant=0.001  UdotUserProvided=0
  Simulink-PS Converter2 : nesl_utility/Simulink-PS Converter  PhysicalDomain=network_engine_domain  SubClassName=ps_input  LeftPortType=input  RightPortType=output  PseudoPeriodic=off  Frequencies=[]  NoiseDistribution=none  NoiseParameters=[]  Unit=N  AffineConversion=off  FilteringAndDerivatives=provide  SimscapeFilterOrder=1  InputFilterTimeConstant=0.001  UdotUserProvided=0
  Simulink-PS Converter3 : nesl_utility/Simulink-PS Converter  PhysicalDomain=network_engine_domain  SubClassName=ps_input  LeftPortType=input  RightPortType=output  PseudoPeriodic=off  Frequencies=[]  NoiseDistribution=none  NoiseParameters=[]  Unit=rad  AffineConversion=off  FilteringAndDerivatives=filter  SimscapeFilterOrder=2  InputFilterTimeConstant=sysParams.Simulation.dt  UdotUserProvided=0
  Simulink-PS Converter4 : nesl_utility/Simulink-PS Converter  PhysicalDomain=network_engine_domain  SubClassName=ps_input  LeftPortType=input  RightPortType=output  PseudoPeriodic=off  Frequencies=[]  NoiseDistribution=none  NoiseParameters=[]  Unit=rad  AffineConversion=off  FilteringAndDerivatives=filter  SimscapeFilterOrder=2  InputFilterTimeConstant=sysParams.Simulation.dt  UdotUserProvided=0
  Simulink-PS Converter5 : nesl_utility/Simulink-PS Converter  PhysicalDomain=network_engine_domain  SubClassName=ps_input  LeftPortType=input  RightPortType=output  PseudoPeriodic=off  Frequencies=[]  NoiseDistribution=none  NoiseParameters=[]  Unit=rad  AffineConversion=off  FilteringAndDerivatives=filter  SimscapeFilterOrder=2  InputFilterTimeConstant=sysParams.Simulation.dt  UdotUserProvided=0
  To Virtual Bus : SignalConversion  ConversionOutput=Virtual bus  OverrideOpt=off
  To Virtual Bus1 : SignalConversion  ConversionOutput=Virtual bus  OverrideOpt=off
  WORLD : PMIOPort  Side=Left
  PLATFORM : PMIOPort  Port=2  Side=Right
  PlatformPHYS_OUT : Outport  OutDataTypeStr=Bus: PHYS_OUT
  wires:
  PS-Simulink Converter/1 -> Bus Assignment/2
  PS-Simulink Converter1/1 -> Bus Assignment/3
  PS-Simulink Converter2/1 -> Bus Assignment/4
  PS-Simulink Converter3/1 -> Bus Assignment/5
  PS-Simulink Converter4/1 -> Bus Assignment/6
  PS-Simulink Converter5/1 -> Bus Assignment/7
  Constant/1 -> Bus Assignment/1
  Bus Assignment/1 -> PlatformPHYS_OUT/1
  PlatformPHYS_IN/1 -> Bus Selector1/1, Bus Selector/1
  Bus Selector/1 -> To Virtual Bus/1  "<baseAcc>"
  TotalMass/1 -> Matrix Multiply1/1
  Matrix Multiply1/1 -> Selector/1, Selector1/1, Selector2/1  "Force"
  Selector1/1 -> Signal Modifier1/1
  Selector2/1 -> Signal Modifier2/1
  Bus to Vector/1 -> Matrix Multiply1/2
  To Virtual Bus/1 -> Bus to Vector/1
  Bus to Vector1/1 -> Integrator3/1  "P Q R"
  Selector3/1 -> Signal Modifier3/1
  Selector4/1 -> Signal Modifier4/1
  Selector5/1 -> Signal Modifier5/1
  Integrator3/1 -> Selector4/1, Selector3/1, Selector5/1
  To Virtual Bus1/1 -> Bus to Vector1/1
  Bus Selector1/1 -> To Virtual Bus1/1  "<baseRates>"
  Selector/1 -> Signal Modifier/1
  Signal Modifier/1 -> Simulink-PS Converter/1
  Signal Modifier1/1 -> Simulink-PS Converter1/1
  Signal Modifier2/1 -> Simulink-PS Converter2/1
  Constant1/1 -> Signal Modifier/3
  Constant2/1 -> Signal Modifier1/3
  Constant3/1 -> Signal Modifier2/3
  Constant4/1 -> Signal Modifier/2
  Constant5/1 -> Signal Modifier1/2
  Constant6/1 -> Signal Modifier2/2
  Signal Modifier3/1 -> Simulink-PS Converter3/1
  Signal Modifier4/1 -> Simulink-PS Converter4/1
  Signal Modifier5/1 -> Simulink-PS Converter5/1
  Constant8/1 -> Signal Modifier3/2
  Constant7/1 -> Signal Modifier3/3
  Constant9/1 -> Signal Modifier5/3
  Constant10/1 -> Signal Modifier5/2
  Constant12/1 -> Signal Modifier4/2
  Constant11/1 -> Signal Modifier4/3
  connections:
  PS-Simulink Converter5/LConn1 -- Platform Interface/RConn7
  PS-Simulink Converter4/LConn1 -- Platform Interface/RConn6
  Platform Interface/RConn5 -- PS-Simulink Converter3/LConn1
  Platform Interface/LConn1 -- WORLD/RConn1
  Platform Interface/RConn1 -- PLATFORM/RConn1
  PS-Simulink Converter/LConn1 -- Platform Interface/RConn2
  Platform Interface/RConn3 -- PS-Simulink Converter1/LConn1
  Platform Interface/RConn4 -- PS-Simulink Converter2/LConn1
  Simulink-PS Converter/RConn1 -- Platform Interface/LConn2
  Simulink-PS Converter1/RConn1 -- Platform Interface/LConn3
  Simulink-PS Converter2/RConn1 -- Platform Interface/LConn4
  Simulink-PS Converter4/RConn1 -- Platform Interface/LConn6
  Simulink-PS Converter3/RConn1 -- Platform Interface/LConn5
  Simulink-PS Converter5/RConn1 -- Platform Interface/LConn7

== system Simscape_Gimbals__Lib/Signal Modifier ==
  sigIn : Inport
  reverseSignFlag : Inport  Port=2
  zeroInpuFlag : Inport  Port=3
  Constant : Constant  Value=0
  Switch : Switch  Criteria=u2 > Threshold  Threshold=0.5  SaturateOnIntegerOverflow=off  InputSameDT=off
  Switch1 : Switch  Criteria=u2 > Threshold  SaturateOnIntegerOverflow=off  InputSameDT=off
  Unary Minus : UnaryMinus
  sigOut : Outport
  wires:
  sigIn/1 -> Unary Minus/1, Switch/3
  Switch/1 -> Switch1/3
  Switch1/1 -> sigOut/1
  Constant/1 -> Switch1/1
  reverseSignFlag/1 -> Switch/2
  Unary Minus/1 -> Switch/1
  zeroInpuFlag/1 -> Switch1/2
